simulink model "simulink1"  (R2024b)
settings: Solver=VariableStepAuto  StartTime=0.0  StopTime=10.0  RelTol=1e-3
settings Model: Creator=muradaliyev  LastModifiedBy=muradaliyev

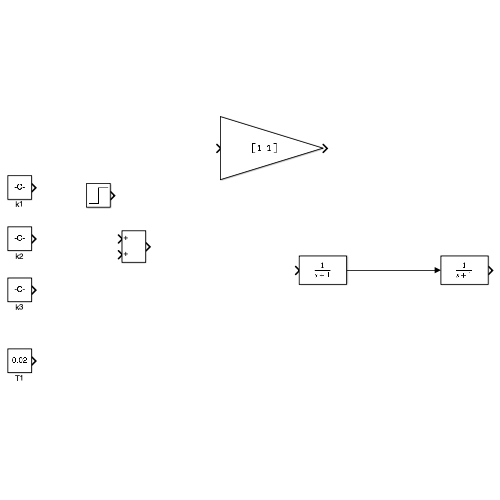
[thumbnail: Simulink's stored preview of the top-level diagram]
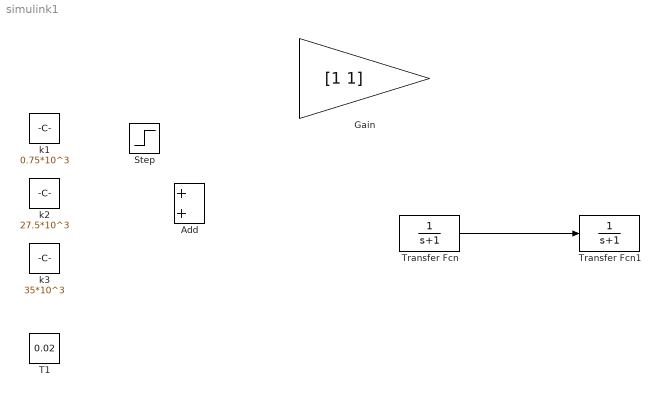
== system simulink1 ==
  Add : Sum
  Gain : Gain  Gain=[1 1]
  Step : Step  SampleTime=0
  T1 : Constant  Value=0.02
  Transfer Fcn : TransferFcn  Denominator=[1 1]
  Transfer Fcn1 : TransferFcn  Denominator=[1 1]
  k1 : Constant  Value=0.75*10^3
  k2 : Constant  Value=27.5*10^3
  k3 : Constant  Value=35*10^3
  wires:
  Transfer Fcn/1 -> Transfer Fcn1/1
